simulink library "tty"  (Simulink 8.1)
settings: Solver=ode1  StartTime=0.0  StopTime=Inf  FixedStep=0.001  RelTol=1e-3
PostLoadFcn:
  | , if any(exist('dsrtsu_mdlpostloadfcn', 'file') == [2, 3, 6]), try dsrtsu_mdlpostloadfcn('Execute', bdroot); catch fprintf('Error in PostLoadFcn (dsrtsu_mdlpostloadfcn) for model "%s":\n %s\n', bdroot, lasterr); end, end,
undefined symbols (not defined in the file or in its folder): ENUM_TARGETTYPE_BICYCLE, ENUM_TARGETTYPE_MOTORBIKE, ENUM_TARGETTYPE_NONE, ENUM_TARGETTYPE_PED, ENUM_TARGETTYPE_TRUCK, ENUM_TARGETTYPE_VEHICLE
settings Model: DSRTSU_INTERNAL_RTI_VER=450  DSRTSU_INTERNAL_RTI_TYPE=rti1401  RTICANMMDATA=struct('GeneralSetupData',struct('modelroot','D:\PROJECTS\HAITEC\TAIWAN_HAITEC_SVN\trunk\AdasDragon\software\sw_development\arch\app\ifo','generalsettings',struct('filesettings',struct('destfolder',struct('Name','RTICANMM_FILES','Check',1),'buildfolder',struct('Name','.','Check',1),'AbsDestfolder',struct('Name','D:\PROJECTS\HAITEC\TAIWAN_HAITEC_SVN\trunk\AdasDragon\software\sw_development\arch\app\ifo\RTICANMM_FILES'),'AbsBuildfolder',struct('Name','D:\PROJECTS\HAITEC\TAIWAN_HAITEC_SVN\trunk\AdasDragon\software\sw_development\arch\app\ifo'))),'options',struct('addpaths',1,'rmpaths',1,'addtrcexclusion',logical(1),'cannavigator',struct('checkmonitoring',0),'show_usrtrc',0,'use_usrtrc',0),'advanced',struct('options',[1 1 1 1 1 1 1 1 1 1 1 1 1 1 1 1 1 1 1 1 1 1 1 1 1 1 1 1 1 1 1 1 1 1 1 1 1 1 1 1 1 1 1 1 1 1 1 1 1 1 1 1 1 1 1 1 1 1 1 1 1 1 1 1 1 1 1 1 1 1 1 1 1 1 1 1 1 1 1 1 1 1 1 1 1 1 1 1 1 1 1 1 1 1 1 1 1 1 1 1]),'MPSetup',{{}},'modelname','tty','block','tty'))  DSRTSU_INTERNAL_RTIFPGA=40  Creator=tescamilla  LastModifiedBy=tescamilla

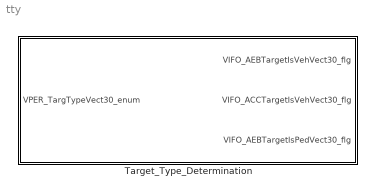
== system tty ==
  Target_Type_Determination : Subsystem

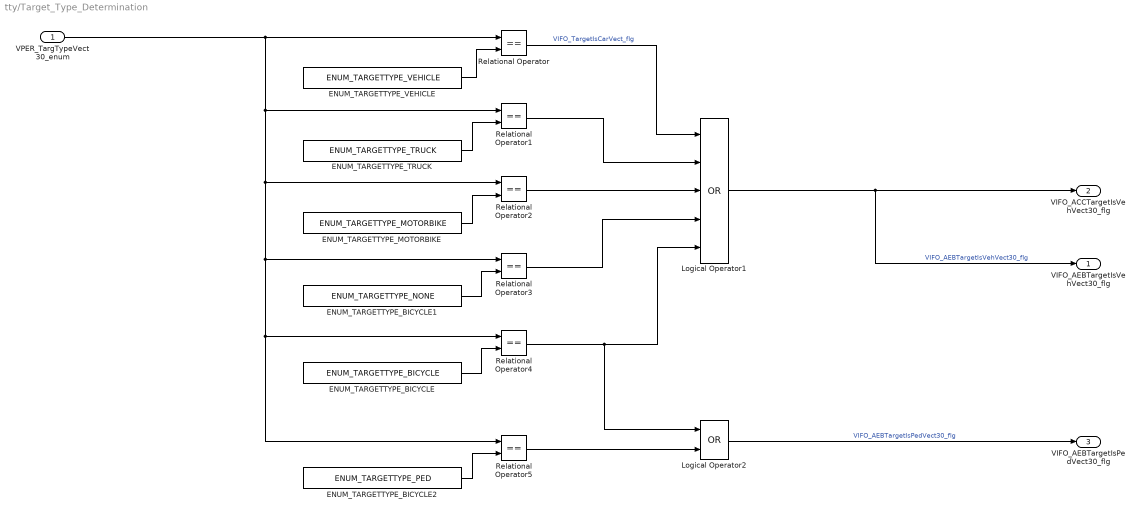
== system tty/Target_Type_Determination ==
  VPER_TargTypeVect30_enum : Inport
  ENUM_TARGETTYPE_BICYCLE : Constant  Value=ENUM_TARGETTYPE_BICYCLE
  ENUM_TARGETTYPE_BICYCLE1 : Constant  Value=ENUM_TARGETTYPE_NONE
  ENUM_TARGETTYPE_BICYCLE2 : Constant  Value=ENUM_TARGETTYPE_PED
  ENUM_TARGETTYPE_MOTORBIKE : Constant  Value=ENUM_TARGETTYPE_MOTORBIKE
  ENUM_TARGETTYPE_TRUCK : Constant  Value=ENUM_TARGETTYPE_TRUCK
  ENUM_TARGETTYPE_VEHICLE : Constant  Value=ENUM_TARGETTYPE_VEHICLE
  Logical Operator1 : Logic  Operator=OR  Inputs=5  AllPortsSameDT=off  OutDataTypeStr=boolean
  Logical Operator2 : Logic  Operator=OR  AllPortsSameDT=off  OutDataTypeStr=boolean
  Relational Operator{,1..5} (6 alike) : RelationalOperator  Operator===  OutDataTypeStr=boolean
  VIFO_AEBTargetIsVehVect30_flg : Outport
  VIFO_ACCTargetIsVehVect30_flg : Outport  Port=2
  VIFO_AEBTargetIsPedVect30_flg : Outport  Port=3
  wires:
  Relational Operator5/1 -> Logical Operator2/2
  ENUM_TARGETTYPE_BICYCLE2/1 -> Relational Operator5/2
  VPER_TargTypeVect30_enum/1 -> Relational Operator1/1, Relational Operator2/1, Relational Operator4/1, Relational Operator5/1, Relational Operator3/1, Relational Operator/1
  Logical Operator2/1 -> VIFO_AEBTargetIsPedVect30_flg/1  "VIFO_AEBTargetIsPedVect30_flg"
  ENUM_TARGETTYPE_BICYCLE/1 -> Relational Operator4/2
  Relational Operator4/1 -> Logical Operator2/1, Logical Operator1/5
  Relational Operator2/1 -> Logical Operator1/3
  ENUM_TARGETTYPE_BICYCLE1/1 -> Relational Operator3/2
  ENUM_TARGETTYPE_MOTORBIKE/1 -> Relational Operator2/2
  Relational Operator1/1 -> Logical Operator1/2
  ENUM_TARGETTYPE_TRUCK/1 -> Relational Operator1/2
  Relational Operator/1 -> Logical Operator1/1  "VIFO_TargetIsCarVect_flg"
  ENUM_TARGETTYPE_VEHICLE/1 -> Relational Operator/2
  Logical Operator1/1 -> VIFO_ACCTargetIsVehVect30_flg/1, VIFO_AEBTargetIsVehVect30_flg/1  "VIFO_AEBTargetIsVehVect30_flg"
  Relational Operator3/1 -> Logical Operator1/4
